simulink model "ex1_sim"  (R2015b)
settings: Solver=ode45  StartTime=0.0  StopTime=simtime  RelTol=1e-3
values from neighbouring files (symbols this model uses):
  D = [0; 0]    [ex1.m]    (also in ex6.m = [0 0; 0 0; 0 0])
  J = (J1 + J2)    (= 3.6e-05)    [ex1.m]    (also in ex2.m; ex3.m)
  motor = motor_pars    [ex1.m]
  sim_V = Vmax    (= 1)    [ex1.m]    (also in ex2.m; ex3.m; ex4.m; ex5.m = 24)
settings Model: Creator=andfro  LastModifiedBy=Lamn
settings DataIOCC: SaveFormat=Array
settings DebuggingCC: SolverPrmCheckMsg=warning
settings HardwareCC: ProdBitPerPointer=32  ProdLargestAtomicFloat=None  ProdIntDivRoundTo=Undefined  ProdEndianess=Unspecified  ProdWordSize=32  ProdHWDeviceType=32-bit Generic
settings GRTTargetCC: GeneratePreprocessorConditionals=Disable all
settings ConfigComp: CovModelRefEnable=Off  CovSFcnEnable=off

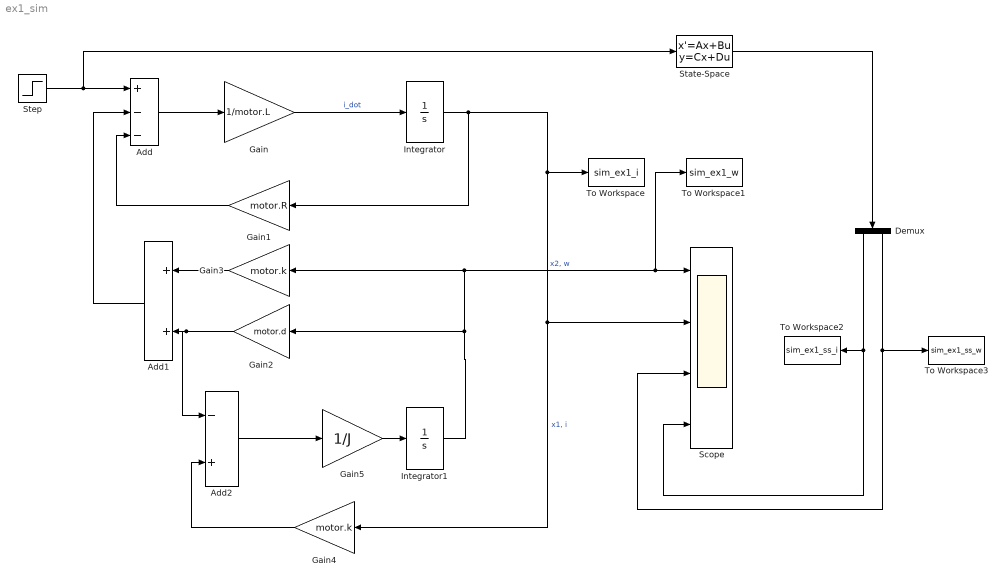
== system ex1_sim ==
  Add : Sum  Inputs=+--
  Add1 : Sum
  Add2 : Sum  Inputs=-+
  Demux : Demux  Outputs=2
  Gain : Gain  Gain=1/motor.L
  Gain1 : Gain  Gain=motor.R
  Gain2 : Gain  Gain=motor.d
  Gain3 : Gain  Gain=motor.k
  Gain4 : Gain  Gain=motor.k
  Gain5 : Gain  Gain=1/J
  Integrator : Integrator
  Integrator1 : Integrator
  Scope : Scope  NumInputPorts=4
  State-Space : StateSpace  A=motor.A  B=motor.B  C=motor.C  D=D  X0=0
  Step : Step  Time=0  After=sim_V  SampleTime=0
  To Workspace : ToWorkspace  VariableName=sim_ex1_i  SaveFormat=Timeseries  SampleTime=-1
  To Workspace1 : ToWorkspace  VariableName=sim_ex1_w  SaveFormat=Timeseries  SampleTime=-1
  To Workspace2 : ToWorkspace  VariableName=sim_ex1_ss_i  SaveFormat=Timeseries  SampleTime=-1
  To Workspace3 : ToWorkspace  VariableName=sim_ex1_ss_w  SaveFormat=Timeseries  SampleTime=-1
  wires:
  Add/1 -> Gain/1
  Step/1 -> State-Space/1, Add/1
  Gain/1 -> Integrator/1  "i_dot"
  Integrator/1 -> Gain1/1, To Workspace/1, Scope/2, Gain4/1  "x1, i"
  Gain1/1 -> Add/3
  Integrator1/1 -> Gain3/1, To Workspace1/1, Scope/1, Gain2/1  "x2, w"
  Gain3/1 -> Add1/1
  Gain2/1 -> Add2/1, Add1/2
  Add1/1 -> Add/2
  Add2/1 -> Gain5/1
  Gain5/1 -> Integrator1/1
  Gain4/1 -> Add2/2
  State-Space/1 -> Demux/1
  Demux/1 -> To Workspace2/1, Scope/4
  Demux/2 -> To Workspace3/1, Scope/3
